simulink model "flightplan2interpreted"  (R2021b)
settings: Solver=VariableStepAuto  StartTime=0.0  StopTime=10.0  RelTol=1e-3
values from neighbouring files (symbols this model uses):
  tabla1 = readtable('SIDs.xlsx')    [creacionestructurasborrador.m]    (also in flight_plan.m = table2struct(tabla1); flight_plan_eval.m = table2struct(tabla1); flight_plan_struct.m = table2struct(tabla1); flight_plan_tabla.m)
  tabla2 = readtable('WPs.xlsx')    [creacionestructurasborrador.m]    (also in flight_plan.m = table2struct(tabla2); flight_plan_eval.m = table2struct(tabla2); flight_plan_struct.m = table2struct(tabla2); tablas.mat = )
  tabla3 = readtable('IAPs.xlsx')    [creacionestructurasborrador.m]    (also in flight_plan.m = table2struct(tabla3); flight_plan_eval.m = table2struct(tabla3); flight_plan_struct.m = table2struct(tabla3); flight_plan_tabla.m)
settings Model: Creator=verti  LastModifiedBy=verti

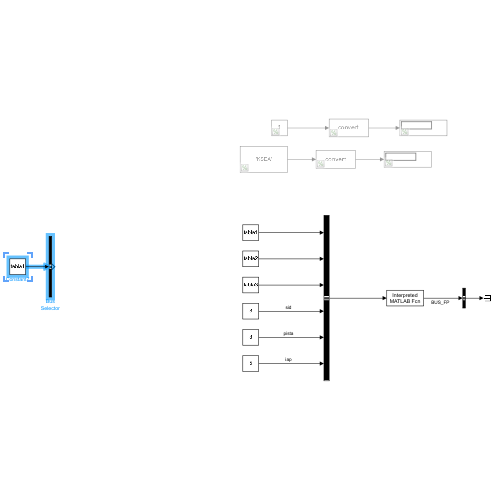
[thumbnail: Simulink's stored preview of the top-level diagram]
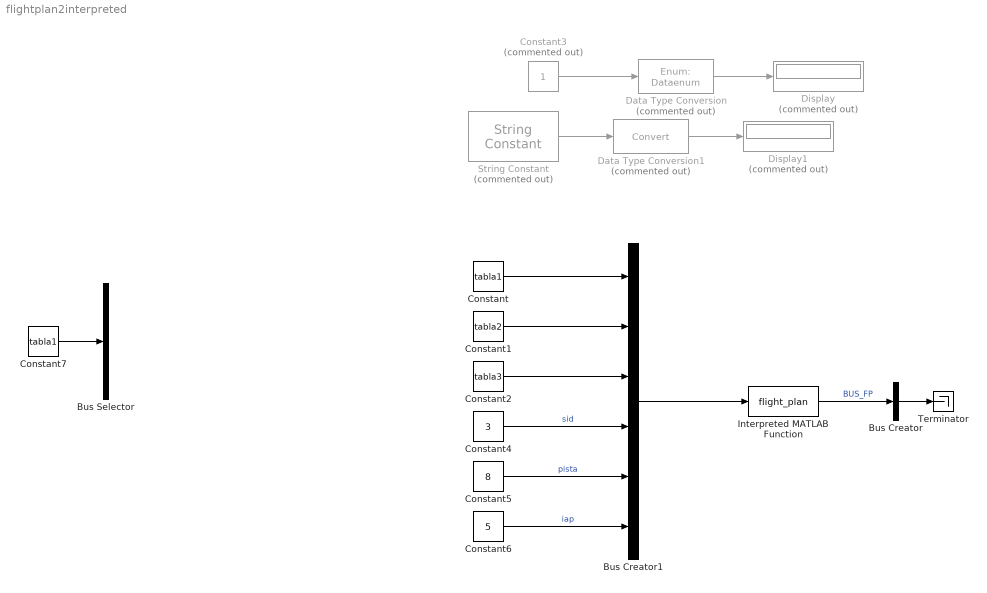
== system flightplan2interpreted ==
  Bus Creator : BusCreator  Inputs=1
  Bus Creator1 : BusCreator  Inputs=6
  Bus Selector : BusSelector  OutputSignals=signal1,signal2,SID,Runway,Latitude,Altitude  OutputAsBus=on
  Constant : Constant  Value=tabla1  OutDataTypeStr=Bus: BUS_SID
  Constant1 : Constant  Value=tabla2  OutDataTypeStr=Bus: BUS_WP
  Constant2 : Constant  Value=tabla3  OutDataTypeStr=Bus: BUS_IAP
  Constant3 : Constant  Commented=on  OutDataTypeStr=int32
  Constant4 : Constant  Value=3
  Constant5 : Constant  Value=8
  Constant6 : Constant  Value=5
  Constant7 : Constant  Value=tabla1  OutDataTypeStr=Bus: BUS_SID
  Data Type Conversion : DataTypeConversion  Commented=on  OutDataTypeStr=Enum: Dataenum
  Data Type Conversion1 : DataTypeConversion  Commented=on
  Display : Display  Commented=on
  Display1 : Display  Commented=on
  Interpreted MATLAB Function : MATLABFcn  MATLABFcn=flight_plan
  String Constant : StringConstant  Commented=on  String='KSEA'
  Terminator : Terminator
  wires:
  Constant3/1 -> Data Type Conversion/1
  Data Type Conversion/1 -> Display/1
  String Constant/1 -> Data Type Conversion1/1
  Data Type Conversion1/1 -> Display1/1
  Constant1/1 -> Bus Creator1/2
  Constant5/1 -> Bus Creator1/5  "pista"
  Constant4/1 -> Bus Creator1/4  "sid"
  Constant2/1 -> Bus Creator1/3
  Interpreted MATLAB Function/1 -> Bus Creator/1  "BUS_FP"
  Constant6/1 -> Bus Creator1/6  "iap"
  Bus Creator/1 -> Terminator/1
  Bus Creator1/1 -> Interpreted MATLAB Function/1
  Constant/1 -> Bus Creator1/1
  Constant7/1 -> Bus Selector/1
